simulink subsystem "Komponovkaobject"  (R2023a)
settings: Solver=VariableStepAuto  StartTime=0.0  StopTime=10.0  RelTol=1e-3
settings Model: Creator=stude  LastModifiedBy=stude

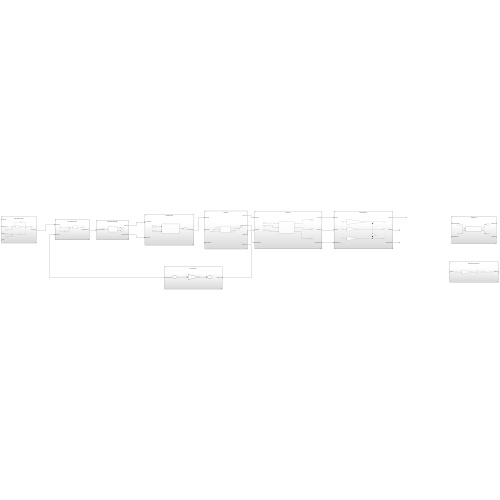
[thumbnail: Simulink's stored preview of the top-level diagram]
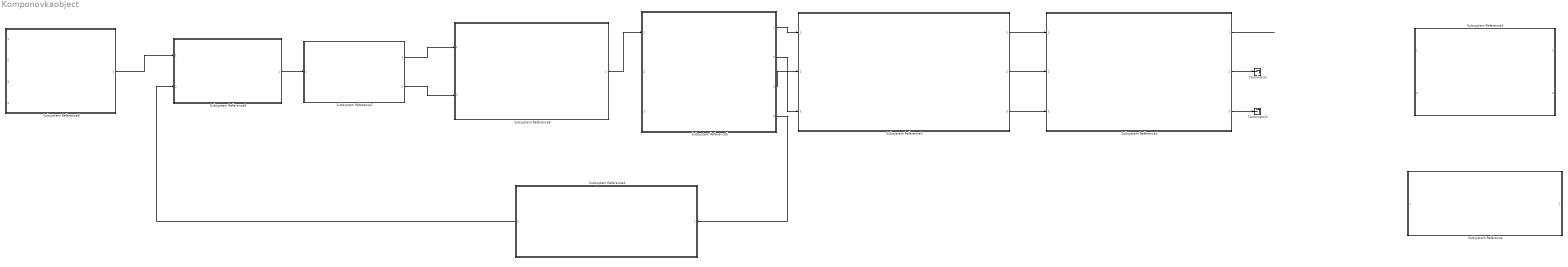
== system Komponovkaobject ==
  Subsystem Reference : Subsystem  ReferencedSubsystem=BackwardAccConverter1
  Subsystem Reference1 : Subsystem  ReferencedSubsystem=HallSensor1
  Subsystem Reference2 : Subsystem  ReferencedSubsystem=RackandPinion1
  Subsystem Reference3 : Subsystem  ReferencedSubsystem=Reductor1
  Subsystem Reference4 : Subsystem  ReferencedSubsystem=CurrentSensor1
  Subsystem Reference5 : Subsystem  ReferencedSubsystem=MOTOR_
  Subsystem Reference6 : Subsystem  ReferencedSubsystem=POWER_GAIN
  Subsystem Reference7 : Subsystem  ReferencedSubsystem=CONTROLADAPTER_
  Subsystem Reference8 : Subsystem  ReferencedSubsystem=HighLevelController
  Subsystem Reference9 : Subsystem  ReferencedSubsystem=LowLevelController1
  Terminator : Terminator
  Terminator1 : Terminator
  wires:
  Subsystem Reference3/1 -> Subsystem Reference2/1
  Subsystem Reference3/2 -> Subsystem Reference2/2
  Subsystem Reference3/3 -> Subsystem Reference2/3
  Subsystem Reference2/2 -> Terminator/1
  Subsystem Reference2/3 -> Terminator1/1
  Subsystem Reference2/1 -> ?
  Subsystem Reference7/1 -> Subsystem Reference6/1
  Subsystem Reference7/2 -> Subsystem Reference6/2
  Subsystem Reference6/1 -> Subsystem Reference5/1
  Subsystem Reference5/1 -> Subsystem Reference3/1
  Subsystem Reference5/2 -> Subsystem Reference3/3
  Subsystem Reference5/3 -> Subsystem Reference3/2
  Subsystem Reference9/1 -> Subsystem Reference7/1
  Subsystem Reference5/4 -> Subsystem Reference4/1
  Subsystem Reference4/1 -> Subsystem Reference9/2
  Subsystem Reference8/1 -> Subsystem Reference9/1
